simulink model "Isc"  (Simulink 8.4)
settings: Solver=ode45  StartTime=0.0  StopTime=10.0  RelTol=1e-3
undefined symbols (not defined in the file): Isc_EngSpdStabLimit, Isc_EngSpdStabOverride, Isc_facEgasMin, Isc_facEngSpdStab, Isc_facIdleSpeedReq, Isc_flgIdleSpeedCtrlEnable, Isc_FuelCutoffDelay, Isc_FuelCutoffEnable, Isc_IdleSpeedReq, Isc_IPartMax, Isc_IPartMaxCatHeat, Isc_IPartMin, Isc_IPartMinCatHeat, Isc_Leerlaufoverride, Isc_rpmIdleCtrlActivMax, Isc_rpmIdleCtrlActivMin
libraries: simulink x2
settings Model: Creator=YAL9FE  LastModifiedBy=ric9fe
settings DebuggingCC: FcnCallInpInsideContextMsg=EnableAllAsWarning

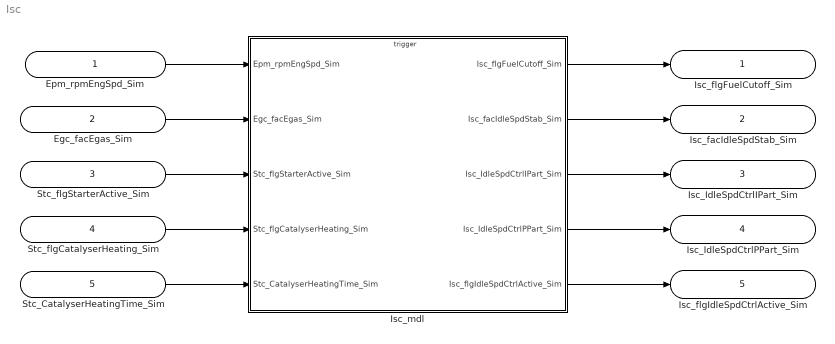
== system Isc ==
  Epm_rpmEngSpd_Sim : Inport
  Egc_facEgas_Sim : Inport  Port=2
  Stc_flgStarterActive_Sim : Inport  Port=3
  Stc_flgCatalyserHeating_Sim : Inport  Port=4
  Stc_CatalyserHeatingTime_Sim : Inport  Port=5
  Isc_mdl : Subsystem  mask(Functions){}
      mask help: IdleSpeedController
      mask Display:
      | image(imread('IdleSpeedController.jpg'))
      | port_label('input',1,'Epm_rpmEngSpd_Sim')
      | port_label('input',2,'Egc_facEgas_Sim')
      | port_label('input',3,'Stc_flgStarterActive_Sim')
      | port_label('input',4,'Stc_flgCatalyserHeating_Sim')
      | port_label('input',5,'Stc_CatalyserHeatingTime_Sim')
      | port_label('output',1,'Isc_flgFuelCutoff_Sim')
      | port_label('output',2,'Isc_facIdleSpdStab_Sim')
      | port_label('output',3,'Isc_IdleSpdCtrlIPart_Sim')
      | port_label('output',4,'Isc_IdleSpdCtrlPPart_Sim')
      | port_label('output',5,'Isc_flgIdleSpdCtrlActive_Sim')
  Isc_flgFuelCutoff_Sim : Outport
  Isc_facIdleSpdStab_Sim : Outport  Port=2
  Isc_IdleSpdCtrlIPart_Sim : Outport  Port=3
  Isc_IdleSpdCtrlPPart_Sim : Outport  Port=4
  Isc_flgIdleSpdCtrlActive_Sim : Outport  Port=5
  wires:
  Epm_rpmEngSpd_Sim/1 -> Isc_mdl/1(Epm_rpmEngSpd_Sim)
  Egc_facEgas_Sim/1 -> Isc_mdl/2(Egc_facEgas_Sim)
  Stc_flgStarterActive_Sim/1 -> Isc_mdl/3(Stc_flgStarterActive_Sim)
  Stc_flgCatalyserHeating_Sim/1 -> Isc_mdl/4(Stc_flgCatalyserHeating_Sim)
  Stc_CatalyserHeatingTime_Sim/1 -> Isc_mdl/5(Stc_CatalyserHeatingTime_Sim)
  Isc_mdl/1(Isc_flgFuelCutoff_Sim) -> Isc_flgFuelCutoff_Sim/1
  Isc_mdl/2(Isc_facIdleSpdStab_Sim) -> Isc_facIdleSpdStab_Sim/1
  Isc_mdl/3(Isc_IdleSpdCtrlIPart_Sim) -> Isc_IdleSpdCtrlIPart_Sim/1
  Isc_mdl/4(Isc_IdleSpdCtrlPPart_Sim) -> Isc_IdleSpdCtrlPPart_Sim/1
  Isc_mdl/5(Isc_flgIdleSpdCtrlActive_Sim) -> Isc_flgIdleSpdCtrlActive_Sim/1

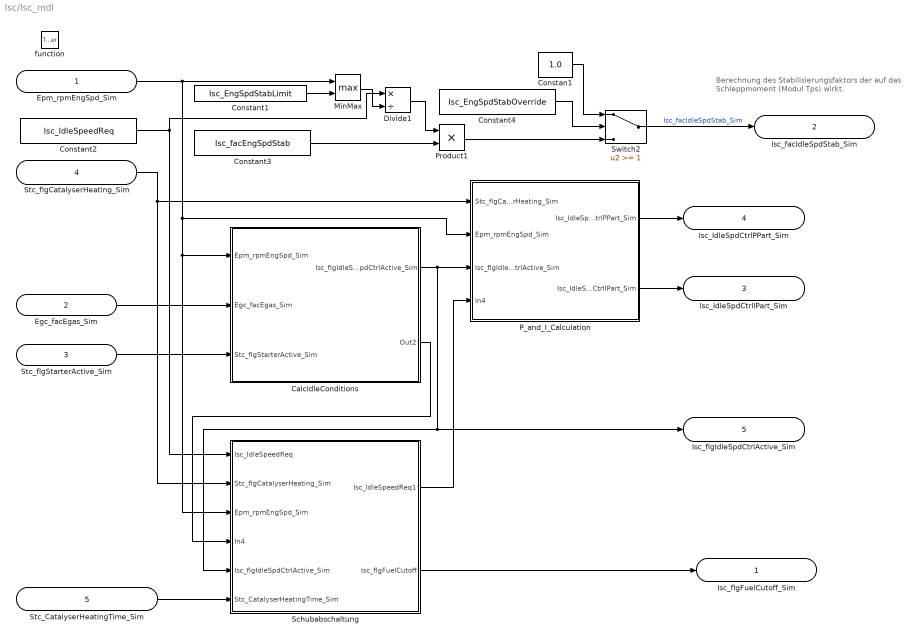
== system Isc/Isc_mdl ==
  note: Berechnung des Stabilisierungsfaktors der auf das Schleppmoment (Modul Tps) wirkt.
  Epm_rpmEngSpd_Sim : Inport
  Egc_facEgas_Sim : Inport  Port=2
  Stc_flgStarterActive_Sim : Inport  Port=3
  Stc_flgCatalyserHeating_Sim : Inport  Port=4
  Stc_CatalyserHeatingTime_Sim : Inport  Port=5
  function : TriggerPort  TriggerType=function-call
  CalcIdleConditions : Subsystem
  Constan1 : Constant  Value=1.0  OutDataTypeStr=single
  Constant1 : Constant  Value=Isc_EngSpdStabLimit
  Constant2 : Constant  Value=Isc_IdleSpeedReq
  Constant3 : Constant  Value=Isc_facEngSpdStab
  Constant4 : Constant  Value=Isc_EngSpdStabOverride
  Divide1 : Product  Inputs=*/  OutDataTypeStr=Inherit: Same as first input
  MinMax : MinMax  Function=max  Inputs=2
  P_and_I_Calculation : Subsystem
  Product1 : Product  OutDataTypeStr=Inherit: Same as first input
  Schubabschaltung : Subsystem
  Switch2 : Switch  Threshold=1
  Isc_flgFuelCutoff_Sim : Outport
  Isc_facIdleSpdStab_Sim : Outport  Port=2
  Isc_IdleSpdCtrlIPart_Sim : Outport  Port=3
  Isc_IdleSpdCtrlPPart_Sim : Outport  Port=4
  Isc_flgIdleSpdCtrlActive_Sim : Outport  Port=5
  wires:
  Constant2/1 -> Divide1/1, Schubabschaltung/1(Isc_IdleSpeedReq)
  MinMax/1 -> Divide1/2
  Constant1/1 -> MinMax/2
  Epm_rpmEngSpd_Sim/1 -> Schubabschaltung/3(Epm_rpmEngSpd_Sim), CalcIdleConditions/1(Epm_rpmEngSpd_Sim), P_and_I_Calculation/2(Epm_rpmEngSpd_Sim), MinMax/1
  Divide1/1 -> Product1/1
  Constant3/1 -> Product1/2
  Product1/1 -> Switch2/3
  Constan1/1 -> Switch2/1
  Constant4/1 -> Switch2/2
  Switch2/1 -> Isc_facIdleSpdStab_Sim/1  "Isc_facIdleSpdStab_Sim"
  Stc_flgCatalyserHeating_Sim/1 -> Schubabschaltung/2(Stc_flgCatalyserHeating_Sim), P_and_I_Calculation/1(Stc_flgCatalyserHeating_Sim)
  CalcIdleConditions/1(Isc_flgIdleSpdCtrlActive_Sim) -> P_and_I_Calculation/3(Isc_flgIdleSpdCtrlActive_Sim), Schubabschaltung/5(Isc_flgIdleSpdCtrlActive_Sim), Isc_flgIdleSpdCtrlActive_Sim/1
  Egc_facEgas_Sim/1 -> CalcIdleConditions/2(Egc_facEgas_Sim)
  Stc_flgStarterActive_Sim/1 -> CalcIdleConditions/3(Stc_flgStarterActive_Sim)
  P_and_I_Calculation/1(Isc_IdleSpdCtrlPPart_Sim) -> Isc_IdleSpdCtrlPPart_Sim/1
  P_and_I_Calculation/2(Isc_IdleSpdCtrlIPart_Sim) -> Isc_IdleSpdCtrlIPart_Sim/1
  CalcIdleConditions/2(Out2) -> Schubabschaltung/4(In4)
  Stc_CatalyserHeatingTime_Sim/1 -> Schubabschaltung/6(Stc_CatalyserHeatingTime_Sim)
  Schubabschaltung/1(Isc_IdleSpeedReq1) -> P_and_I_Calculation/4(In4)
  Schubabschaltung/2(Isc_flgFuelCutoff) -> Isc_flgFuelCutoff_Sim/1

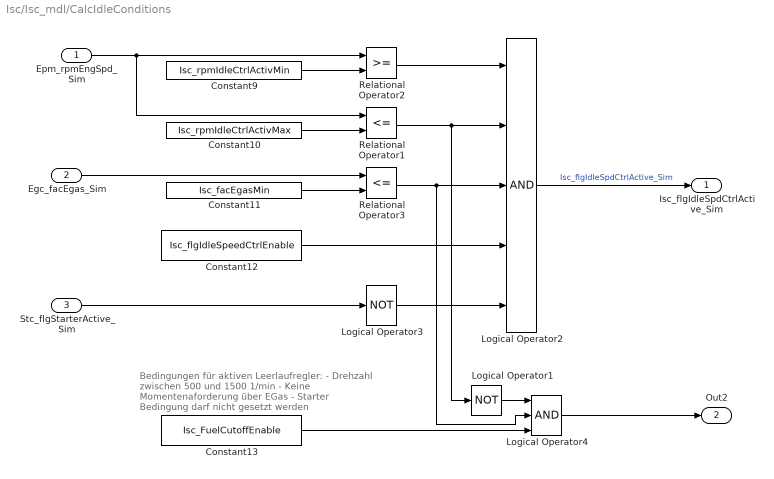
== system Isc/Isc_mdl/CalcIdleConditions ==
  note: Bedingungen für aktiven Leerlaufregler:
      | - Drehzahl zwischen 500 und 1500 1/min
      | - Keine Momentenaforderung über EGas
      | - Starter Bedingung darf nicht gesetzt werden
  Epm_rpmEngSpd_Sim : Inport
  Egc_facEgas_Sim : Inport  Port=2
  Stc_flgStarterActive_Sim : Inport  Port=3
  Constant10 : Constant  Value=Isc_rpmIdleCtrlActivMax
  Constant11 : Constant  Value=Isc_facEgasMin
  Constant12 : Constant  Value=Isc_flgIdleSpeedCtrlEnable
  Constant13 : Constant  Value=Isc_FuelCutoffEnable
  Constant9 : Constant  Value=Isc_rpmIdleCtrlActivMin
  Logical Operator1 : Logic  Operator=NOT  AllPortsSameDT=off  OutDataTypeStr=boolean
  Logical Operator2 : Logic  Inputs=5  AllPortsSameDT=off  OutDataTypeStr=boolean
  Logical Operator3 : Logic  Operator=NOT  AllPortsSameDT=off  OutDataTypeStr=boolean
  Logical Operator4 : Logic  Inputs=3  AllPortsSameDT=off  OutDataTypeStr=boolean
  Relational Operator1 : RelationalOperator  Operator=<=  OutDataTypeStr=boolean
  Relational Operator2 : RelationalOperator  OutDataTypeStr=boolean
  Relational Operator3 : RelationalOperator  Operator=<=  OutDataTypeStr=boolean
  Isc_flgIdleSpdCtrlActive_Sim : Outport
  Out2 : Outport  Port=2
  wires:
  Epm_rpmEngSpd_Sim/1 -> Relational Operator1/1, Relational Operator2/1
  Relational Operator2/1 -> Logical Operator2/1
  Constant13/1 -> Logical Operator4/3
  Logical Operator2/1 -> Isc_flgIdleSpdCtrlActive_Sim/1  "Isc_flgIdleSpdCtrlActive_Sim"
  Logical Operator4/1 -> Out2/1
  Stc_flgStarterActive_Sim/1 -> Logical Operator3/1
  Logical Operator1/1 -> Logical Operator4/1
  Constant12/1 -> Logical Operator2/4
  Constant10/1 -> Relational Operator1/2
  Relational Operator1/1 -> Logical Operator2/2, Logical Operator1/1
  Egc_facEgas_Sim/1 -> Relational Operator3/1
  Constant11/1 -> Relational Operator3/2
  Logical Operator3/1 -> Logical Operator2/5
  Relational Operator3/1 -> Logical Operator2/3, Logical Operator4/2
  Constant9/1 -> Relational Operator2/2

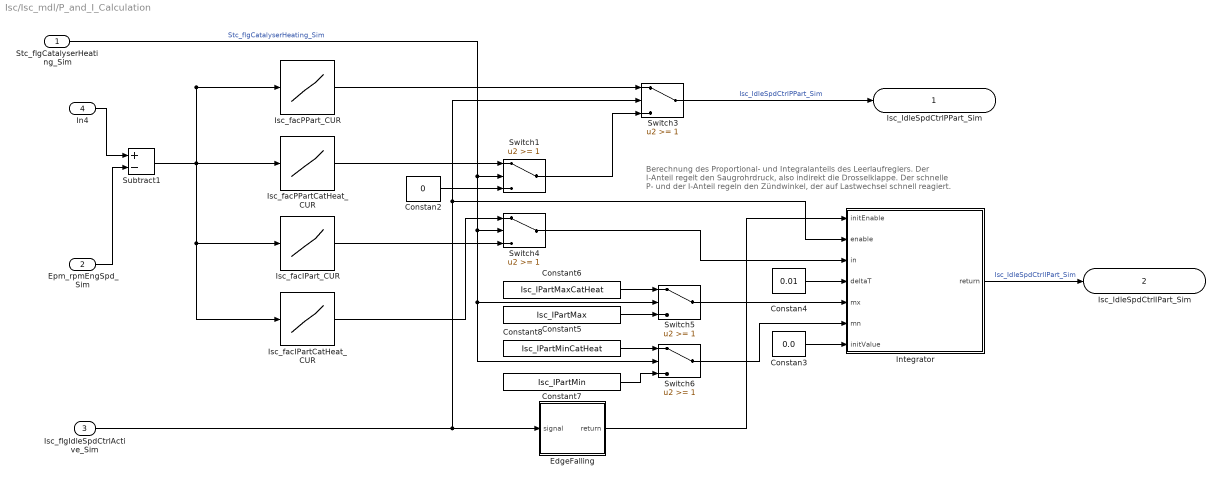
== system Isc/Isc_mdl/P_and_I_Calculation ==
  note: Berechnung des Proportional- und Integralanteils des Leerlaufreglers.
      | Der I-Anteil regelt den Saugrohrdruck, also indirekt die Drosselklappe.
      | Der schnelle P- und der I-Anteil regeln den Zündwinkel, der auf
      | Lastwechsel schnell reagiert.
  Stc_flgCatalyserHeating_Sim : Inport
  Epm_rpmEngSpd_Sim : Inport  Port=2
  Isc_flgIdleSpdCtrlActive_Sim : Inport  Port=3
  In4 : Inport  Port=4
  Constan2 : Constant  Value=0  OutDataTypeStr=single
  Constan3 : Constant  Value=0.0  OutDataTypeStr=single
  Constan4 : Constant  Value=0.01  OutDataTypeStr=single
  Constant5 : Constant  Value=Isc_IPartMax
  Constant6 : Constant  Value=Isc_IPartMaxCatHeat
  Constant7 : Constant  Value=Isc_IPartMin
  Constant8 : Constant  Value=Isc_IPartMinCatHeat
  EdgeFalling : Subsystem
      mask help: EdgeFalling
      mask Display: image(imread('EdgeFalling.jpg'))
  Integrator : Subsystem
      mask help: Integrator
      mask Display: image(imread('Integrator.jpg'))
  Isc_facIPartCatHeat_CUR : Lookup_n-D  NumberOfTableDimensions=1  BreakpointsForDimension1=[1:3]  Table=[10 18 23]  ExtrapMethod=Clip  InputSameDT=on
  Isc_facIPart_CUR : Lookup_n-D  NumberOfTableDimensions=1  BreakpointsForDimension1=[1:3]  Table=[16 19 20]  ExtrapMethod=Clip  InputSameDT=on
  Isc_facPPartCatHeat_CUR : Lookup_n-D  NumberOfTableDimensions=1  BreakpointsForDimension1=[1:3]  Table=[4 5 6]  ExtrapMethod=Clip  InputSameDT=on
  Isc_facPPart_CUR : Lookup_n-D  NumberOfTableDimensions=1  BreakpointsForDimension1=[1:3]  Table=[10 18 23]  ExtrapMethod=Clip  InputSameDT=on
  Subtract1 : Sum  Inputs=+-  OutDataTypeStr=Inherit: Same as first input
  Switch{1,3..6} (5 alike) : Switch  Threshold=1
  Isc_IdleSpdCtrlPPart_Sim : Outport
  Isc_IdleSpdCtrlIPart_Sim : Outport  Port=2
  wires:
  Isc_flgIdleSpdCtrlActive_Sim/1 -> EdgeFalling/1(signal), Switch3/2, Integrator/2(enable)
  Stc_flgCatalyserHeating_Sim/1 -> Switch1/2, Switch4/2, Switch5/2, Switch6/2  "Stc_flgCatalyserHeating_Sim"
  Epm_rpmEngSpd_Sim/1 -> Subtract1/2
  Subtract1/1 -> Isc_facPPart_CUR/1, Isc_facPPartCatHeat_CUR/1, Isc_facIPart_CUR/1, Isc_facIPartCatHeat_CUR/1
  Constan2/1 -> Switch1/3
  Switch1/1 -> Switch3/3
  Switch3/1 -> Isc_IdleSpdCtrlPPart_Sim/1  "Isc_IdleSpdCtrlPPart_Sim"
  Isc_facPPartCatHeat_CUR/1 -> Switch1/1
  Isc_facPPart_CUR/1 -> Switch3/1
  Integrator/1(return) -> Isc_IdleSpdCtrlIPart_Sim/1  "Isc_IdleSpdCtrlIPart_Sim"
  Isc_facIPart_CUR/1 -> Switch4/3
  Isc_facIPartCatHeat_CUR/1 -> Switch4/1
  Switch4/1 -> Integrator/3(in)
  Constan3/1 -> Integrator/7(initValue)
  Constan4/1 -> Integrator/4(deltaT)
  Switch5/1 -> Integrator/5(mx)
  Switch6/1 -> Integrator/6(mn)
  Constant6/1 -> Switch5/1
  Constant5/1 -> Switch5/3
  Constant8/1 -> Switch6/1
  Constant7/1 -> Switch6/3
  EdgeFalling/1(return) -> Integrator/1(initEnable)
  In4/1 -> Subtract1/1

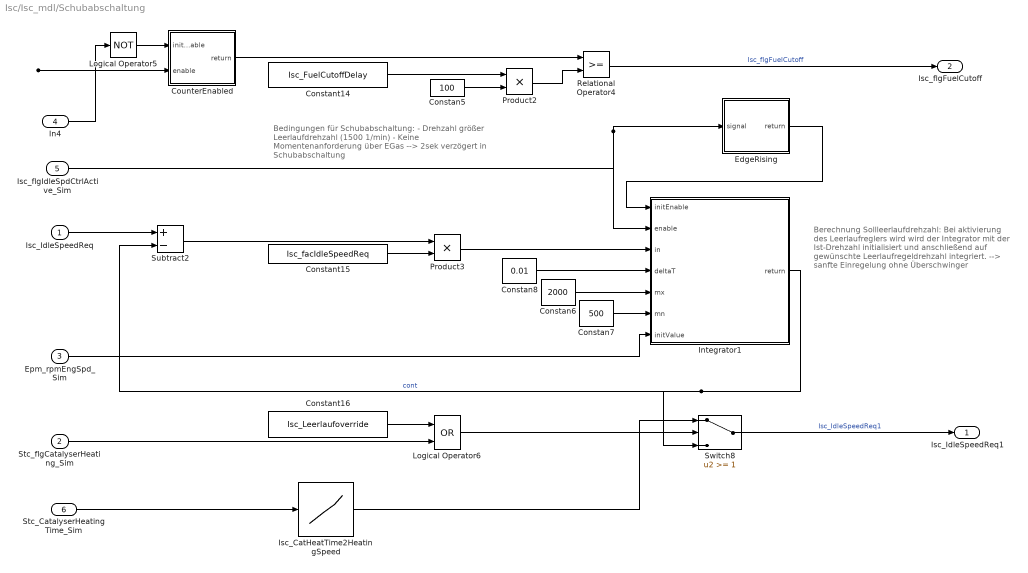
== system Isc/Isc_mdl/Schubabschaltung ==
  note: Bedingungen für Schubabschaltung:
      | - Drehzahl größer Leerlaufdrehzahl (1500 1/min)
      | - Keine Momentenanforderung über EGas
      | --> 2sek verzögert in Schubabschaltung
  note: Berechnung Sollleerlaufdrehzahl:
      | Bei aktivierung des Leerlaufreglers wird
      | wird der Integrator mit der Ist-Drehzahl
      | initialisiert und anschließend auf gewünschte
      | Leerlaufregeldrehzahl integriert.
      | --> sanfte Einregelung ohne Überschwinger
  Isc_IdleSpeedReq : Inport
  Stc_flgCatalyserHeating_Sim : Inport  Port=2
  Epm_rpmEngSpd_Sim : Inport  Port=3
  In4 : Inport  Port=4
  Isc_flgIdleSpdCtrlActive_Sim : Inport  Port=5
  Stc_CatalyserHeatingTime_Sim : Inport  Port=6
  Constan5 : Constant  Value=100  OutDataTypeStr=single
  Constan6 : Constant  Value=2000  OutDataTypeStr=single
  Constan7 : Constant  Value=500  OutDataTypeStr=single
  Constan8 : Constant  Value=0.01  OutDataTypeStr=single
  Constant14 : Constant  Value=Isc_FuelCutoffDelay
  Constant15 : Constant  Value=Isc_facIdleSpeedReq
  Constant16 : Constant  Value=Isc_Leerlaufoverride
  CounterEnabled : Subsystem
      mask help: Counter
      mask Display: image(imread('CounterEnabled.jpg'))
  EdgeRising : Subsystem
      mask help: EdgeRising
      mask Display: image(imread('EdgeRising.jpg'))
  Integrator1 : Subsystem
      mask help: Integrator
      mask Display: image(imread('Integrator.jpg'))
  Isc_CatHeatTime2HeatingSpeed : Lookup_n-D  NumberOfTableDimensions=1  BreakpointsForDimension1=[1:3]  Table=[13 19 20]  ExtrapMethod=Clip  InputSameDT=on
  Logical Operator5 : Logic  Operator=NOT  AllPortsSameDT=off  OutDataTypeStr=boolean
  Logical Operator6 : Logic  Operator=OR  AllPortsSameDT=off  OutDataTypeStr=boolean
  Product2 : Product  OutDataTypeStr=Inherit: Same as first input
  Product3 : Product  OutDataTypeStr=Inherit: Same as first input
  Relational Operator4 : RelationalOperator  OutDataTypeStr=boolean
  Subtract2 : Sum  Inputs=+-  OutDataTypeStr=Inherit: Same as first input
  Switch8 : Switch  Threshold=1
  Isc_IdleSpeedReq1 : Outport
  Isc_flgFuelCutoff : Outport  Port=2
  wires:
  Switch8/1 -> Isc_IdleSpeedReq1/1  "Isc_IdleSpeedReq1"
  Epm_rpmEngSpd_Sim/1 -> Integrator1/7(initValue)
  Stc_flgCatalyserHeating_Sim/1 -> Logical Operator6/2
  Isc_IdleSpeedReq/1 -> Subtract2/1
  Isc_flgIdleSpdCtrlActive_Sim/1 -> EdgeRising/1(signal), Integrator1/2(enable)
  Logical Operator5/1 -> CounterEnabled/1(initEnable)
  CounterEnabled/1(return) -> Relational Operator4/1
  Product2/1 -> Relational Operator4/2
  Constant14/1 -> Product2/1
  Constan5/1 -> Product2/2
  Relational Operator4/1 -> Isc_flgFuelCutoff/1  "Isc_flgFuelCutoff"
  Subtract2/1 -> Product3/1
  Constant15/1 -> Product3/2
  Product3/1 -> Integrator1/3(in)
  EdgeRising/1(return) -> Integrator1/1(initEnable)
  Constan8/1 -> Integrator1/4(deltaT)
  Constan6/1 -> Integrator1/5(mx)
  Constan7/1 -> Integrator1/6(mn)
  Integrator1/1(return) -> Subtract2/2, Switch8/3  "cont"
  Constant16/1 -> Logical Operator6/1
  Logical Operator6/1 -> Switch8/2
  Stc_CatalyserHeatingTime_Sim/1 -> Isc_CatHeatTime2HeatingSpeed/1
  Isc_CatHeatTime2HeatingSpeed/1 -> Switch8/1
  In4/1 -> Logical Operator5/1, CounterEnabled/2(enable)

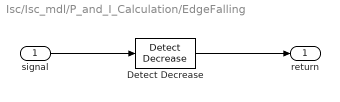
== system Isc/Isc_mdl/P_and_I_Calculation/EdgeFalling ==
  signal : Inport
  Detect Decrease : simulink/Logic and Bit Operations/Detect Decrease  vinit=0.0  InputProcessing=Inherited  OutDataTypeStr=boolean
  return : Outport
  wires:
  Detect Decrease/1 -> return/1
  signal/1 -> Detect Decrease/1

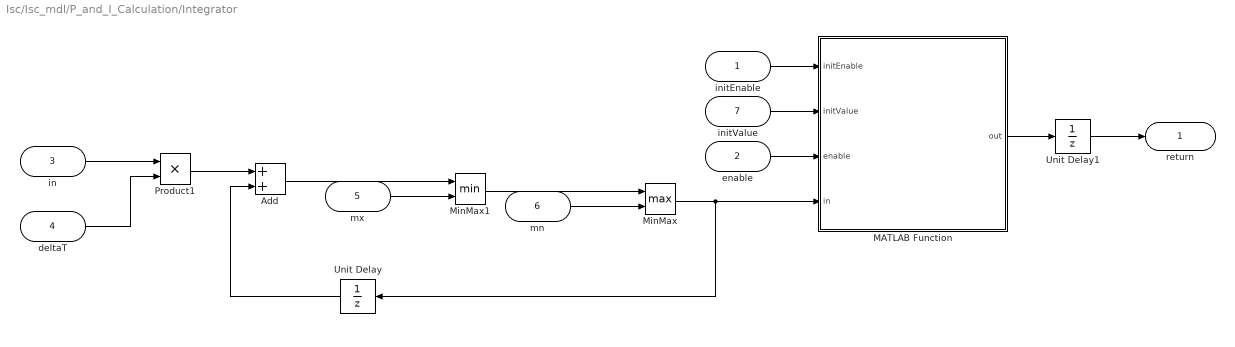
== system Isc/Isc_mdl/P_and_I_Calculation/Integrator ==
  initEnable : Inport
  enable : Inport  Port=2
  in : Inport  Port=3
  deltaT : Inport  Port=4
  mx : Inport  Port=5
  mn : Inport  Port=6
  initValue : Inport  Port=7
  Add : Sum
  MATLAB Function : MATLAB Function  TreatAsAtomicUnit=on
  MinMax : MinMax  Function=max  Inputs=2
  MinMax1 : MinMax  Inputs=2
  Product1 : Product  OutDataTypeStr=Inherit: Same as first input
  Unit Delay : UnitDelay  SampleTime=-1
  Unit Delay1 : UnitDelay  SampleTime=-1
  return : Outport
  wires:
  deltaT/1 -> Product1/2
  in/1 -> Product1/1
  Product1/1 -> Add/1
  Add/1 -> MinMax1/1
  mx/1 -> MinMax1/2
  MinMax1/1 -> MinMax/1
  mn/1 -> MinMax/2
  Unit Delay/1 -> Add/2
  MinMax/1 -> Unit Delay/1, MATLAB Function/4(in)
  MATLAB Function/1(out) -> Unit Delay1/1
  enable/1 -> MATLAB Function/3(enable)
  initValue/1 -> MATLAB Function/2(initValue)
  initEnable/1 -> MATLAB Function/1(initEnable)
  Unit Delay1/1 -> return/1

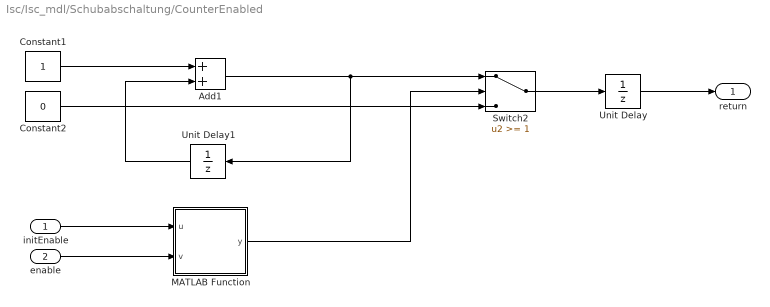
== system Isc/Isc_mdl/Schubabschaltung/CounterEnabled ==
  initEnable : Inport
  enable : Inport  Port=2
  Add1 : Sum
  Constant1 : Constant  OutDataTypeStr=single
  Constant2 : Constant  Value=0  OutDataTypeStr=single
  MATLAB Function : MATLAB Function  TreatAsAtomicUnit=on
  Switch2 : Switch  Threshold=1
  Unit Delay : UnitDelay  SampleTime=-1
  Unit Delay1 : UnitDelay  SampleTime=-1
  return : Outport
  wires:
  initEnable/1 -> MATLAB Function/1(u)
  MATLAB Function/1(y) -> Switch2/2
  Add1/1 -> Unit Delay1/1, Switch2/1
  Constant2/1 -> Switch2/3
  Switch2/1 -> Unit Delay/1
  Unit Delay1/1 -> Add1/2
  Constant1/1 -> Add1/1
  enable/1 -> MATLAB Function/2(v)
  Unit Delay/1 -> return/1

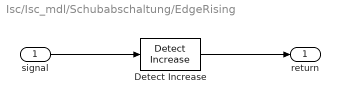
== system Isc/Isc_mdl/Schubabschaltung/EdgeRising ==
  signal : Inport
  Detect Increase : simulink/Logic and Bit Operations/Detect Increase  vinit=0.0  InputProcessing=Inherited  OutDataTypeStr=boolean
  return : Outport
  wires:
  Detect Increase/1 -> return/1
  signal/1 -> Detect Increase/1

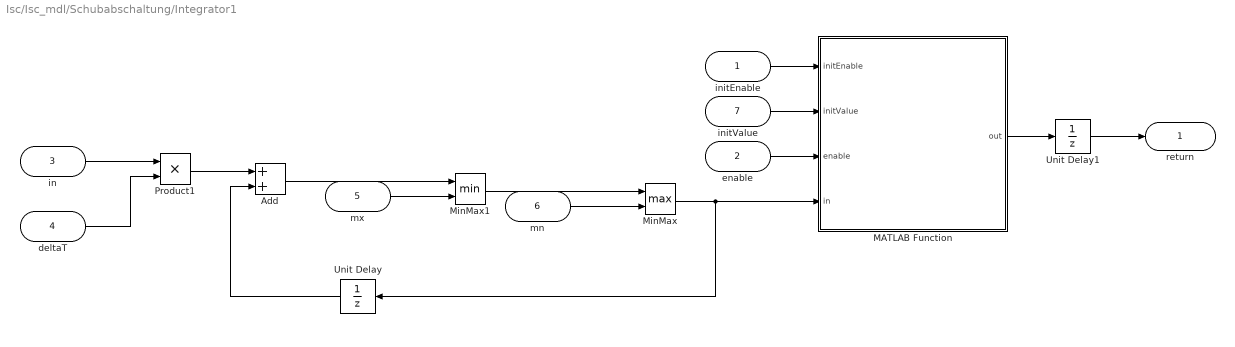
== system Isc/Isc_mdl/Schubabschaltung/Integrator1 ==
  initEnable : Inport
  enable : Inport  Port=2
  in : Inport  Port=3
  deltaT : Inport  Port=4
  mx : Inport  Port=5
  mn : Inport  Port=6
  initValue : Inport  Port=7
  Add : Sum
  MATLAB Function : MATLAB Function  TreatAsAtomicUnit=on
  MinMax : MinMax  Function=max  Inputs=2
  MinMax1 : MinMax  Inputs=2
  Product1 : Product  OutDataTypeStr=Inherit: Same as first input
  Unit Delay : UnitDelay  SampleTime=-1
  Unit Delay1 : UnitDelay  SampleTime=-1
  return : Outport
  wires:
  Unit Delay1/1 -> return/1
  initEnable/1 -> MATLAB Function/1(initEnable)
  initValue/1 -> MATLAB Function/2(initValue)
  enable/1 -> MATLAB Function/3(enable)
  MATLAB Function/1(out) -> Unit Delay1/1
  MinMax/1 -> MATLAB Function/4(in), Unit Delay/1
  Unit Delay/1 -> Add/2
  mn/1 -> MinMax/2
  MinMax1/1 -> MinMax/1
  mx/1 -> MinMax1/2
  Add/1 -> MinMax1/1
  Product1/1 -> Add/1
  in/1 -> Product1/1
  deltaT/1 -> Product1/2

== matlab function Isc_mdl/P_and_I_Calculation/Integrator/MATLAB Function ==
  data: initEnable input double; out output double; initValue input double; enable input double; in input double
function out = fcn(initEnable,initValue,enable,in)
% Integrator Test
out = single(0.0);
if(initEnable==true)
    out = initValue;
end
if(enable==true)
    out = single(in);
end

== matlab function Isc_mdl/Schubabschaltung/CounterEnabled/MATLAB Function ==
  data: u input double; y output double; v input double
function y = fcn(u,v)
% CounterEnabled Test
y = false;
if(u==true)
    y = false;
end
if(v==true)
    y = true;
end

== matlab function Isc_mdl/Schubabschaltung/Integrator1/MATLAB Function ==
  data: initEnable input double; out output double; initValue input double; enable input double; in input double
function out = fcn(initEnable,initValue,enable,in)
% Integrator Test
out = single(0.0);
if(initEnable==true)
    out = initValue;
end
if(enable==true)
    out = single(in);
end
